simulink model "ssp_ad_preaddr"  (Simulink 6.5)
settings: Solver=VariableStepDiscrete  SolverMode=SingleTasking  StartTime=0.0  StopTime=100  RelTol=1e-3
undefined symbols (not defined in the file or in its folder): sigbuilder_block
libraries: xbsIndex_r4 x12, nort_sysgenlib x1
settings Model: Creator=nort  LastModifiedBy=nort

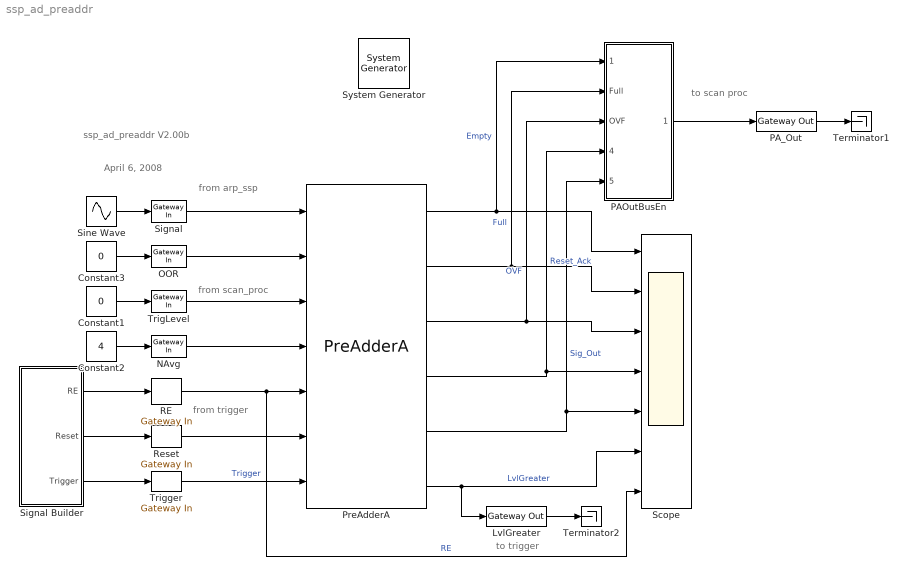
== system ssp_ad_preaddr ==
  note: ssp_ad_preaddr V2.00b
  note: April 6, 2008
  note: from arp_ssp
  note: from scan_proc
  note: from trigger
  note: to scan proc
  note: to trigger
  " System Generator" : xbsIndex_r4/ System Generator  Tag=genX  SystemSampleTime=-1  xilinxfamily=virtex4  part=xc4vlx25  speed=-10  package=ff668  synthesis_tool=XST  directory=./pa_netlist  testbench=off  simulink_period=1  sysclk_period=10  incr_netlist=off  trim_vbits=Everywhere in SubSystem  dbl_ovrd=According to Block Masks  core_generation=According to Block Masks  run_coregen=off  deprecated_control=off  eval_field=0  block_type=sysgen
      settings: block_version=9.1.01
  Constant1 : Constant  Value=0  OutDataType=sfix(16)  ConRadixGroup=Use specified scaling  OutScaling=2^0  SampleTime=inf  FramePeriod=inf
  Constant2 : Constant  Value=4  OutDataType=sfix(16)  ConRadixGroup=Use specified scaling  OutScaling=2^0  SampleTime=inf  FramePeriod=inf
  Constant3 : Constant  Value=0  OutDataType=sfix(16)  ConRadixGroup=Use specified scaling  OutScaling=2^0  SampleTime=inf  FramePeriod=inf
  LvlGreater : xbsIndex_r4/Gateway Out  hdl_port=on  timing_constraint=None  locs_specified=off  LOCs={}  block_type=gatewayout
      settings: infoedit="Gateway out block.  Converts Xilinx fixed point inputs into ouputs of type Simulink integer, double, or fixed point.<P><P>Hardware notes:  In hardware these blocks become top level output ports or are discarded, depending on how they are configured."
  NAvg : xbsIndex_r4/Gateway In  arith_type=Unsigned  n_bits=8  bin_pt=0  quantization="Round  (unbiased: +/- Inf)"  overflow=Saturate  period=1  dbl_ovrd=off  timing_constraint=None  locs_specified=off  LOCs={}  block_type=gatewayin
      settings: infoedit="Gateway in block.  Converts inputs of type Simulink integer, double and fixed point to  Xilinx fixed point type.<P><P>Hardware notes:  In hardware these blocks become top level input ports."
  OOR : xbsIndex_r4/Gateway In  arith_type=Boolean  n_bits=1  bin_pt=0  quantization="Round  (unbiased: +/- Inf)"  overflow=Saturate  period=1  dbl_ovrd=off  timing_constraint=None  locs_specified=off  LOCs={}  block_type=gatewayin
      settings: infoedit="Gateway in block.  Converts inputs of type Simulink integer, double and fixed point to  Xilinx fixed point type.<P><P>Hardware notes:  In hardware these blocks become top level input ports."
  PAOutBusEn : Subsystem
  PA_Out : xbsIndex_r4/Gateway Out  hdl_port=on  timing_constraint=None  locs_specified=off  LOCs={}  block_type=gatewayout
      settings: infoedit="Gateway out block.  Converts Xilinx fixed point inputs into ouputs of type Simulink integer, double, or fixed point.<P><P>Hardware notes:  In hardware these blocks become top level output ports or are discarded, depending on how they are configured."
  PreAdderA : nort_sysgenlib/PreAdderA  SystemSampleTime=-1
  RE : xbsIndex_r4/Gateway In  arith_type=Unsigned  n_bits=3  bin_pt=0  quantization="Round  (unbiased: +/- Inf)"  overflow=Saturate  period=1  dbl_ovrd=off  timing_constraint=None  locs_specified=off  LOCs={}  block_type=gatewayin
      settings: infoedit="Gateway in block.  Converts inputs of type Simulink integer, double and fixed point to  Xilinx fixed point type.<P><P>Hardware notes:  In hardware these blocks become top level input ports."  block_version=9.2.01
  Reset : xbsIndex_r4/Gateway In  arith_type=Boolean  n_bits=16  bin_pt=14  quantization="Round  (unbiased: +/- Inf)"  overflow=Saturate  period=1  dbl_ovrd=off  timing_constraint=None  locs_specified=off  LOCs={}  block_type=gatewayin
      settings: infoedit="Gateway in block.  Converts inputs of type Simulink integer, double and fixed point to  Xilinx fixed point type.<P><P>Hardware notes:  In hardware these blocks become top level input ports."  block_version=9.2.01
  Scope : Scope  NumInputPorts=7
      settings: YMin=-5~-5~-5~-5~-5~-5~-5  YMax=5~5~5~5~5~5~5
  Signal : xbsIndex_r4/Gateway In  arith_type="Signed  (2's comp)"  n_bits=16  bin_pt=0  quantization="Round  (unbiased: +/- Inf)"  overflow=Saturate  period=1  dbl_ovrd=off  timing_constraint=None  locs_specified=off  LOCs={}  block_type=gatewayin
      settings: infoedit="Gateway in block.  Converts inputs of type Simulink integer, double and fixed point to  Xilinx fixed point type.<P><P>Hardware notes:  In hardware these blocks become top level input ports."
  Signal Builder : Subsystem  Tag=STV Subsys  LoadFcn=sigbuilder_block('load');  StartFcn=sigbuilder_block('start');  StopFcn=sigbuilder_block('stop');  ClipboardFcn=sigbuilder_block('clipboard');  mask(Sigbuilder block){}
      mask help: Sigbuilder GUI
      mask init:
      | if ~strcmp(get_param(bdroot(gcbh),'SimulationStatus'),'stopped') tuvar = sigbuilder_block('maskInit'); end
      settings: CopyFcn=sigbuilder_block('copy');  DeleteFcn=sigbuilder_block('delete');  ModelCloseFcn=sigbuilder_block('modelClose');  PreSaveFcn=sigbuilder_block('preSave');  NameChangeFcn=sigbuilder_block('namechange');  OpenFcn=sigbuilder_block('open',[190.5 42 550.5 399.75 ]);  CloseFcn=sigbuilder_block('close');
      mask Display: plot(0,0,100,100,[10,10,40,40,10],[80,20,20,80,80],[40,10],[50,50], [40,27,10],[65,72,56],[40,25,25,10],[28,28,43,43]);
  Sine Wave : Sin  SineType=Sample based  Amplitude=30000  Samples=100  SampleTime=[1 0]
  Terminator1 : Terminator
  Terminator2 : Terminator
  TrigLevel : xbsIndex_r4/Gateway In  arith_type="Signed  (2's comp)"  n_bits=16  bin_pt=0  quantization="Round  (unbiased: +/- Inf)"  overflow=Saturate  period=1  dbl_ovrd=off  timing_constraint=None  locs_specified=off  LOCs={}  block_type=gatewayin
      settings: infoedit="Gateway in block.  Converts inputs of type Simulink integer, double and fixed point to  Xilinx fixed point type.<P><P>Hardware notes:  In hardware these blocks become top level input ports."
  Trigger : xbsIndex_r4/Gateway In  arith_type=Boolean  n_bits=1  bin_pt=0  quantization="Round  (unbiased: +/- Inf)"  overflow=Saturate  period=1  dbl_ovrd=off  timing_constraint=None  locs_specified=off  LOCs={}  block_type=gatewayin
      settings: infoedit="Gateway in block.  Converts inputs of type Simulink integer, double and fixed point to  Xilinx fixed point type.<P><P>Hardware notes:  In hardware these blocks become top level input ports."
  wires:
  NAvg/1 -> PreAdderA/4
  Sine Wave/1 -> Signal/1
  Constant2/1 -> NAvg/1
  RE/1 -> Scope/7, PreAdderA/5  "RE"
  LvlGreater/1 -> Terminator2/1
  Reset/1 -> PreAdderA/6
  Trigger/1 -> PreAdderA/7  "Trigger"
  Signal Builder/2(Reset) -> Reset/1
  Signal Builder/3(Trigger) -> Trigger/1
  Signal Builder/1(RE) -> RE/1
  TrigLevel/1 -> PreAdderA/3
  Constant1/1 -> TrigLevel/1
  PreAdderA/5 -> Scope/5, PAOutBusEn/5(Sig_Out)  "Sig_Out"
  Signal/1 -> PreAdderA/1
  PreAdderA/6 -> LvlGreater/1, Scope/6  "LvlGreater"
  PreAdderA/4 -> Scope/4, PAOutBusEn/4(Reset_Ack)  "Reset_Ack"
  PreAdderA/3 -> Scope/3, PAOutBusEn/3(OVF)  "OVF"
  PreAdderA/2 -> Scope/2, PAOutBusEn/2(Full)  "Full"
  PreAdderA/1 -> Scope/1, PAOutBusEn/1(Empty)  "Empty"
  PA_Out/1 -> Terminator1/1
  PAOutBusEn/1(PA_Out) -> PA_Out/1
  Constant3/1 -> OOR/1
  OOR/1 -> PreAdderA/2

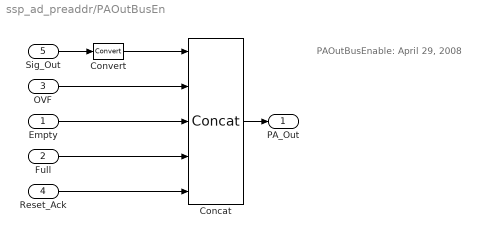
== system ssp_ad_preaddr/PAOutBusEn ==
  note: PAOutBusEnable: April 29, 2008
  Empty : Inport
  Full : Inport  Port=2
  OVF : Inport  Port=3
  Reset_Ack : Inport  Port=4
  Sig_Out : Inport  Port=5
  Concat : xbsIndex_r4/Concat  num_inputs=5  dbl_ovrd=off  block_type=concat
      settings: block_version=9.2.01
  Convert : xbsIndex_r4/Convert  arith_type=Unsigned  n_bits=25  bin_pt=0  quantization=Truncate  overflow=Wrap  latency=0  dbl_ovrd=off  pipeline=off  block_type=convert
      settings: block_version=9.2.01
  PA_Out : Outport
  wires:
  Empty/1 -> Concat/3
  Full/1 -> Concat/4
  OVF/1 -> Concat/2
  Reset_Ack/1 -> Concat/5
  Concat/1 -> PA_Out/1
  Sig_Out/1 -> Convert/1
  Convert/1 -> Concat/1

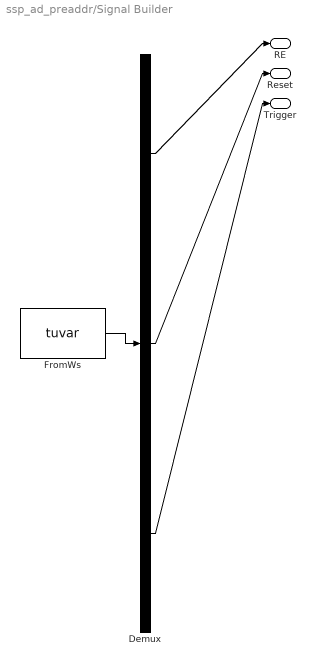
== system ssp_ad_preaddr/Signal Builder ==
  Demux : Demux  Tag=STV Demux  Outputs=3
  FromWs : FromWorkspace  Tag=STV FromWs  VariableName=tuvar  SampleTime=0  SigBuilderData=DataTag1  VnvData=DataTag2
      SigBuilderData=|
      | channels(1).label = 'RE'
      | channels(1).allXData = {[0 19.8 19.8 29 29 31 31 34 34 41 41 44 44 100], [0 5 10 15 20 20 25 25 30 30 35 35 40 40 45 45 50 50 55 55 60 65 70 70 75 75 80 80 85 85 90 90 95 95 100]}
      | channels(1).allYData = {[1 1 2 2 4 4 1 1 2 2 4 4 1 1], [0 0 0 0 0 1 1 0 0 1 1 0 0 1 1 0 0 1 1 0 0 0 0 1 1 0 0 1 1 0 0 1 1 0 0]}
      | channels(2).label = 'Reset'
      | channels(2).allXData = {[0 2 2 4 4 100], [0 2 2 4 4 100]}
      | channels(2).allYData = {[0 0 1 1 0 0], [0 0 1 1 0 0]}
      | channels(3).label = 'Trigger'
      | channels(3).allXData = {[0 12.5 12.5 13.5 13.5 62.5 62.5 63.5 63.5 100], [0 12.5 12.5 13.5 13.5 58.5 58.5 60 60 100]}
      | channels(3).allYData = {[0 0 1 1 0 0 1 1 0 0], [0 0 1 1 0 0 1 1 0 0]}
      | common.afterFinalStr = 'Extrapolate'
      | common.sampleTime = 0
      | dataSet(1).timeRange = [0 100]
      | dataSet(1).name = 'Group 1'
      | dataSet(2).timeRange = [0 100]
      | dataSet(2).name = 'Group 2'
  RE : Outport  Tag=STV Outport
  Reset : Outport  Tag=STV Outport  Port=2
  Trigger : Outport  Tag=STV Outport  Port=3
  wires:
  FromWs/1 -> Demux/1
  Demux/1 -> RE/1
  Demux/2 -> Reset/1
  Demux/3 -> Trigger/1
